simulink model "DAC_test_bench"  (R2017b)
settings: Solver=VariableStepAuto  StartTime=0.0  StopTime=1  RelTol=1e-3
libraries: simulink x1
settings Model: Creator=ucagu  LastModifiedBy=ucagu

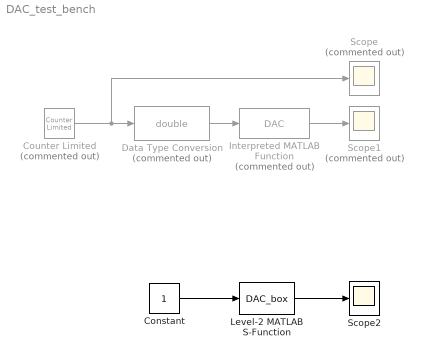
== system DAC_test_bench ==
  Constant : Constant
  Counter Limited : simulink/Sources/Counter Limited  Commented=on  uplimit=256  tsamp=1
  Data Type Conversion : DataTypeConversion  Commented=on  OutDataTypeStr=double
  Interpreted MATLAB Function : MATLABFcn  Commented=on  MATLABFcn=DAC
  Level-2 MATLAB S-Function : M-S-Function  FunctionName=DAC_box  Parameters=1
  Scope : Scope  Commented=on
  Scope1 : Scope  Commented=on
  Scope2 : Scope
  wires:
  Counter Limited/1 -> Data Type Conversion/1, Scope/1
  Data Type Conversion/1 -> Interpreted MATLAB Function/1
  Interpreted MATLAB Function/1 -> Scope1/1
  Constant/1 -> Level-2 MATLAB S-Function/1
  Level-2 MATLAB S-Function/1 -> Scope2/1
